simulink model "CRPNeuralNetwrok"  (R2019b)
settings: Solver=ode45  StartTime=0.0  StopTime=5  FixedStep=0.01  MaxStep=0.05  RelTol=1e-3
settings Model: Creator=user  LastModifiedBy=xyh
settings SolverCC: AlgebraicLoopSolver=LineSearch

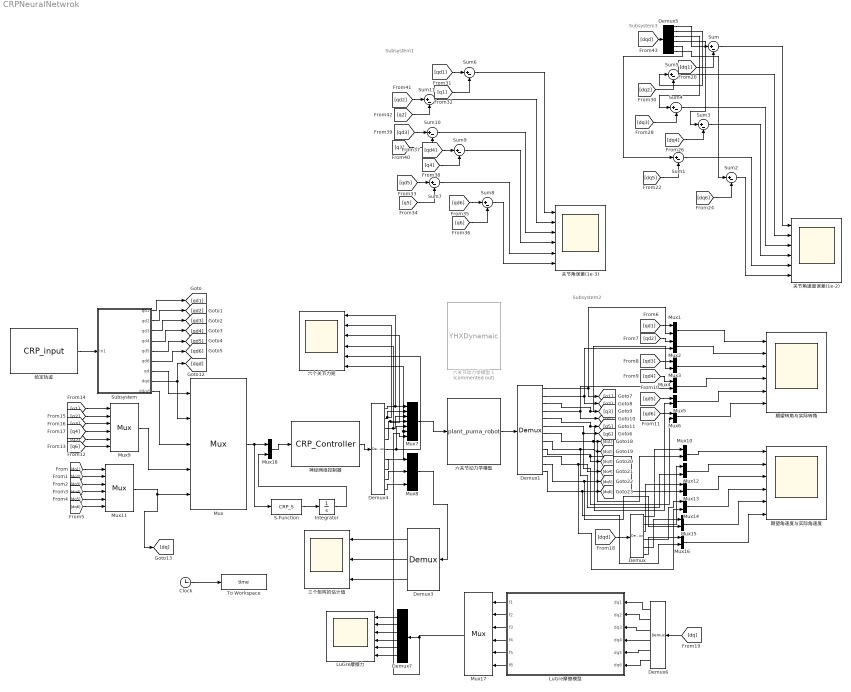
== system CRPNeuralNetwrok ==
  note: Subsystem1
  note: Subsystem3
  note: Subsystem2
  Clock : Clock
  Demux{,5..7} (4 alike) : Demux  Outputs=6
  Demux1 : Demux  Outputs=12
  Demux3 : Demux  Outputs=3
  Demux4 : Demux  Outputs=9
  Integrator : Integrator
  LuGre摩擦力 : Scope  NumInputPorts=6
  LuGre摩擦模型 : Subsystem
  Mux : Mux  Inputs=5
  Mux{1..6,10,12..16,18} (13 alike) : Mux  Inputs=2
  Mux11 : Mux  Inputs=6
  Mux17 : Mux  Inputs=6
  Mux7 : Mux  Inputs=7
  Mux8 : Mux  Inputs=3
  Mux9 : Mux  Inputs=6
  S-Function : S-Function  FunctionName=CRP_S  SFunctionDeploymentMode=off  EnableBusSupport=off
  Subsystem : Subsystem  TreatAsAtomicUnit=on
  Sum{,1..11} (12 alike) : Sum  Inputs=|+-
  To Workspace : ToWorkspace  VariableName=time  SaveFormat=Timeseries  SampleTime=-1
  三个矩阵的估计值 : Scope  NumInputPorts=3
  六个关节力矩 : Scope  NumInputPorts=6
  "六关节动力学模型 " : S-Function  FunctionName=plant_puma_robot  SFunctionDeploymentMode=off  EnableBusSupport=off
  六关节动力学模型 1 : S-Function  Commented=on  FunctionName=YHXDynamaic  SFunctionDeploymentMode=off  EnableBusSupport=off
  关节角误差(1e-3) : Scope  NumInputPorts=6
  关节角速度误差(1e-2) : Scope  NumInputPorts=6
  期望角速度与实际角速度 : Scope  NumInputPorts=6
  期望转角与实际转角 : Scope  NumInputPorts=6
  神经网络控制器 : S-Function  FunctionName=CRP_Controller  SFunctionDeploymentMode=off  EnableBusSupport=off
  给定轨迹 : S-Function  FunctionName=CRP_input  SFunctionDeploymentMode=off  EnableBusSupport=off
  wires:
  Mux7/1 -> "六关节动力学模型 "/1
  Clock/1 -> To Workspace/1
  [dq1] -> Mux11/1
  [dq4] -> Mux11/4
  [dq2] -> Mux11/2
  [dq3] -> Mux11/3
  [dq5] -> Mux11/5
  [dq6] -> Mux11/6
  Demux3/1 -> 三个矩阵的估计值/1
  Demux3/2 -> 三个矩阵的估计值/2
  Demux3/3 -> 三个矩阵的估计值/3
  神经网络控制器/1 -> Demux4/1
  Mux8/1 -> Demux3/1
  [q1] -> Mux9/1
  [q2] -> Mux9/2
  [q3] -> Mux9/3
  [q4] -> Mux9/4
  [q5] -> Mux9/5
  [q6] -> Mux9/6
  "六关节动力学模型 "/1 -> Demux1/1
  Demux4/3 -> 六个关节力矩/4, Mux7/3
  Demux4/1 -> 六个关节力矩/1, Mux7/1
  Demux4/2 -> 六个关节力矩/2, Mux7/2
  Demux4/4 -> 六个关节力矩/3, Mux7/4
  Demux4/5 -> 六个关节力矩/5, Mux7/5
  Demux4/6 -> 六个关节力矩/6, Mux7/6
  Demux4/7 -> Mux8/1
  Demux4/8 -> Mux8/2
  Demux4/9 -> Mux8/3
  Mux/1 -> S-Function/1, Mux18/1
  Mux11/1 -> [dq], Mux/5
  Mux9/1 -> Mux/4
  给定轨迹/1 -> Subsystem/1(In1)
  Subsystem/7(qd) -> Mux/1
  Subsystem/8(dqd) -> [dqd], Mux/2
  Subsystem/9(ddqd) -> Mux/3
  Subsystem/1(qd1) -> [qd1]
  Subsystem/2(qd2) -> [qd2]
  Subsystem/3(qd3) -> [qd3]
  Subsystem/4(qd4) -> [qd4]
  Subsystem/5(qd5) -> [qd5]
  Subsystem/6(qd6) -> [qd6]
  Sum6/1 -> 关节角误差(1e-3)/1
  Sum11/1 -> 关节角误差(1e-3)/2
  Sum10/1 -> 关节角误差(1e-3)/3
  Sum9/1 -> 关节角误差(1e-3)/4
  Sum7/1 -> 关节角误差(1e-3)/5
  Sum8/1 -> 关节角误差(1e-3)/6
  Mux1/1 -> 期望转角与实际转角/1
  Mux2/1 -> 期望转角与实际转角/2
  Mux3/1 -> 期望转角与实际转角/3
  Mux4/1 -> 期望转角与实际转角/4
  Mux5/1 -> 期望转角与实际转角/5
  Mux6/1 -> 期望转角与实际转角/6
  Mux10/1 -> 期望角速度与实际角速度/1
  Mux12/1 -> 期望角速度与实际角速度/2
  Mux13/1 -> 期望角速度与实际角速度/3
  Mux14/1 -> 期望角速度与实际角速度/4
  Mux15/1 -> 期望角速度与实际角速度/5
  Mux16/1 -> 期望角速度与实际角速度/6
  Demux/4 -> Mux14/1
  Demux1/12 -> Mux16/2, [dq6]
  Demux1/2 -> [q2], Mux2/2
  [qd2] -> Mux2/1
  Demux1/4 -> Mux4/2, [q4]
  [qd1] -> Mux1/1
  Demux/3 -> Mux13/1
  Demux1/1 -> [q1], Mux1/2
  Demux/6 -> Mux16/1
  Demux1/10 -> Mux14/2, [dq4]
  Demux/5 -> Mux15/1
  Demux/1 -> Mux10/1
  Demux1/9 -> Mux13/2, [dq3]
  [dqd] -> Demux/1
  [qd6] -> Mux6/1
  Demux1/7 -> Mux10/2, [dq1]
  [qd3] -> Mux3/1
  Demux1/11 -> [dq5], Mux15/2
  [qd4] -> Mux4/1
  [qd5] -> Mux5/1
  Demux1/5 -> Mux5/2, [q5]
  Demux/2 -> Mux12/1
  Demux1/6 -> Mux6/2, [q6]
  Demux1/8 -> Mux12/2, [dq2]
  Demux1/3 -> Mux3/2, [q3]
  Sum/1 -> 关节角速度误差(1e-2)/1
  Sum5/1 -> 关节角速度误差(1e-2)/2
  Sum4/1 -> 关节角速度误差(1e-2)/3
  Sum3/1 -> 关节角速度误差(1e-2)/4
  Sum1/1 -> 关节角速度误差(1e-2)/5
  Sum2/1 -> 关节角速度误差(1e-2)/6
  [dq2] -> Sum5/2
  Demux5/4 -> Sum3/1
  Demux5/5 -> Sum1/1
  Demux5/3 -> Sum4/1
  [dq5] -> Sum1/2
  Demux5/1 -> Sum/1
  [dq6] -> Sum2/2
  Demux5/6 -> Sum2/1
  Demux5/2 -> Sum5/1
  [dq3] -> Sum4/2
  [dq4] -> Sum3/2
  [dq1] -> Sum/2
  [q5] -> Sum7/2
  [qd1] -> Sum6/1
  [qd2] -> Sum11/1
  [q4] -> Sum9/2
  [qd3] -> Sum10/1
  [qd4] -> Sum9/1
  [q3] -> Sum10/2
  [qd5] -> Sum7/1
  [q6] -> Sum8/2
  [qd6] -> Sum8/1
  [q2] -> Sum11/2
  [q1] -> Sum6/2
  [dqd] -> Demux5/1
  LuGre摩擦模型/1(f1) -> Mux17/1
  LuGre摩擦模型/2(f2) -> Mux17/2
  LuGre摩擦模型/3(f3) -> Mux17/3
  LuGre摩擦模型/4(f4) -> Mux17/4
  LuGre摩擦模型/5(f5) -> Mux17/5
  LuGre摩擦模型/6(f6) -> Mux17/6
  [dq] -> Demux6/1
  Demux6/1 -> LuGre摩擦模型/1(dq1)
  Demux6/2 -> LuGre摩擦模型/2(dq2)
  Demux6/3 -> LuGre摩擦模型/3(dq3)
  Demux6/4 -> LuGre摩擦模型/4(dq4)
  Demux6/5 -> LuGre摩擦模型/5(dq5)
  Demux6/6 -> LuGre摩擦模型/6(dq6)
  Mux17/1 -> Mux7/7, Demux7/1
  Demux7/1 -> LuGre摩擦力/1
  Demux7/3 -> LuGre摩擦力/3
  Demux7/4 -> LuGre摩擦力/4
  Demux7/5 -> LuGre摩擦力/5
  Demux7/6 -> LuGre摩擦力/6
  Demux7/2 -> LuGre摩擦力/2
  S-Function/1 -> Integrator/1
  Mux18/1 -> 神经网络控制器/1
  Integrator/1 -> Mux18/2

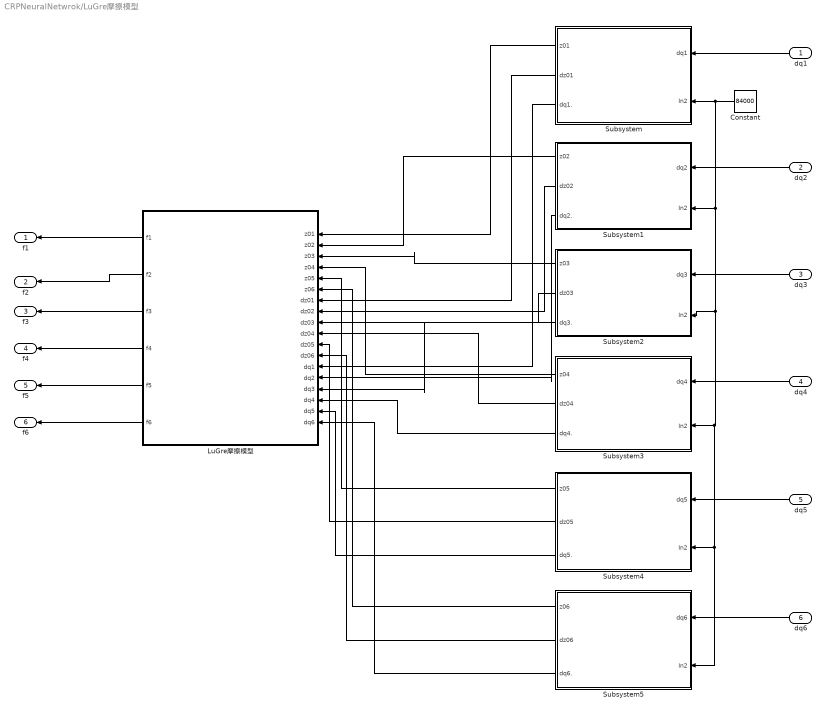
== system CRPNeuralNetwrok/LuGre摩擦模型 ==
  dq1 : Inport
  dq2 : Inport  Port=2
  dq3 : Inport  Port=3
  dq4 : Inport  Port=4
  dq5 : Inport  Port=5
  dq6 : Inport  Port=6
  Constant : Constant  Value=84000
  LuGre摩擦模型 : MATLAB Function  TreatAsAtomicUnit=on
  Subsystem : Subsystem
  Subsystem1 : Subsystem
  Subsystem2 : Subsystem
  Subsystem3 : Subsystem
  Subsystem4 : Subsystem
  Subsystem5 : Subsystem
  f1 : Outport
  f2 : Outport  Port=2
  f3 : Outport  Port=3
  f4 : Outport  Port=4
  f5 : Outport  Port=5
  f6 : Outport  Port=6
  wires:
  LuGre摩擦模型/2(f2) -> f2/1
  LuGre摩擦模型/1(f1) -> f1/1
  Constant/1 -> Subsystem5/2(In2), Subsystem4/2(In2), Subsystem3/2(In2), Subsystem2/2(In2), Subsystem1/2(In2), Subsystem/2(In2)
  dq1/1 -> Subsystem/1(dq1)
  Subsystem/1(z01) -> LuGre摩擦模型/1(z01)
  Subsystem/2(dz01) -> LuGre摩擦模型/7(dz01)
  Subsystem/3(dq1.) -> LuGre摩擦模型/13(dq1)
  dq2/1 -> Subsystem1/1(dq2)
  dq3/1 -> Subsystem2/1(dq3)
  dq4/1 -> Subsystem3/1(dq4)
  dq5/1 -> Subsystem4/1(dq5)
  dq6/1 -> Subsystem5/1(dq6)
  Subsystem1/1(z02) -> LuGre摩擦模型/2(z02)
  Subsystem1/2(dz02) -> LuGre摩擦模型/8(dz02)
  Subsystem1/3(dq2.) -> LuGre摩擦模型/14(dq2)
  Subsystem2/1(z03) -> LuGre摩擦模型/3(z03)
  Subsystem2/2(dz03) -> LuGre摩擦模型/9(dz03)
  Subsystem2/3(dq3.) -> LuGre摩擦模型/15(dq3)
  Subsystem3/1(z04) -> LuGre摩擦模型/4(z04)
  Subsystem3/2(dz04) -> LuGre摩擦模型/10(dz04)
  Subsystem3/3(dq4.) -> LuGre摩擦模型/16(dq4)
  Subsystem4/1(z05) -> LuGre摩擦模型/5(z05)
  Subsystem4/2(dz05) -> LuGre摩擦模型/11(dz05)
  Subsystem4/3(dq5.) -> LuGre摩擦模型/17(dq5)
  Subsystem5/1(z06) -> LuGre摩擦模型/6(z06)
  Subsystem5/2(dz06) -> LuGre摩擦模型/12(dz06)
  Subsystem5/3(dq6.) -> LuGre摩擦模型/18(dq6)
  LuGre摩擦模型/6(f6) -> f6/1
  LuGre摩擦模型/5(f5) -> f5/1
  LuGre摩擦模型/4(f4) -> f4/1
  LuGre摩擦模型/3(f3) -> f3/1

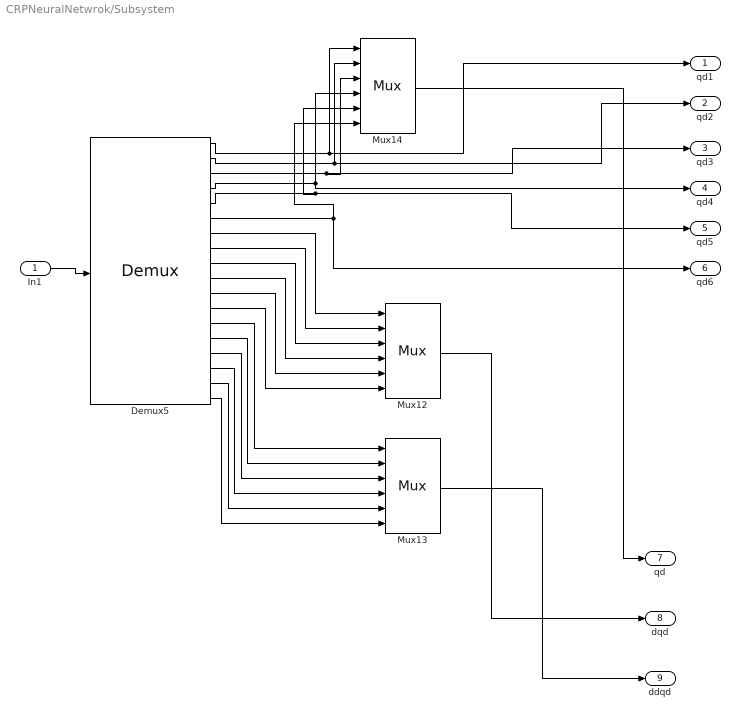
== system CRPNeuralNetwrok/Subsystem ==
  In1 : Inport
  Demux5 : Demux  Outputs=18
  Mux12 : Mux  Inputs=6
  Mux13 : Mux  Inputs=6
  Mux14 : Mux  Inputs=6
  qd1 : Outport
  qd2 : Outport  Port=2
  qd3 : Outport  Port=3
  qd4 : Outport  Port=4
  qd5 : Outport  Port=5
  qd6 : Outport  Port=6
  qd : Outport  Port=7
  dqd : Outport  Port=8
  ddqd : Outport  Port=9
  wires:
  Demux5/8 -> Mux12/2
  Demux5/2 -> Mux14/2, qd2/1
  Demux5/3 -> Mux14/3, qd3/1
  Mux13/1 -> ddqd/1
  Demux5/11 -> Mux12/5
  Demux5/4 -> qd4/1, Mux14/4
  Demux5/1 -> Mux14/1, qd1/1
  Demux5/5 -> Mux14/5, qd5/1
  Demux5/13 -> Mux13/1
  In1/1 -> Demux5/1
  Demux5/7 -> Mux12/1
  Demux5/6 -> Mux14/6, qd6/1
  Mux12/1 -> dqd/1
  Demux5/12 -> Mux12/6
  Demux5/14 -> Mux13/2
  Demux5/18 -> Mux13/6
  Demux5/16 -> Mux13/4
  Mux14/1 -> qd/1
  Demux5/17 -> Mux13/5
  Demux5/10 -> Mux12/4
  Demux5/9 -> Mux12/3
  Demux5/15 -> Mux13/3

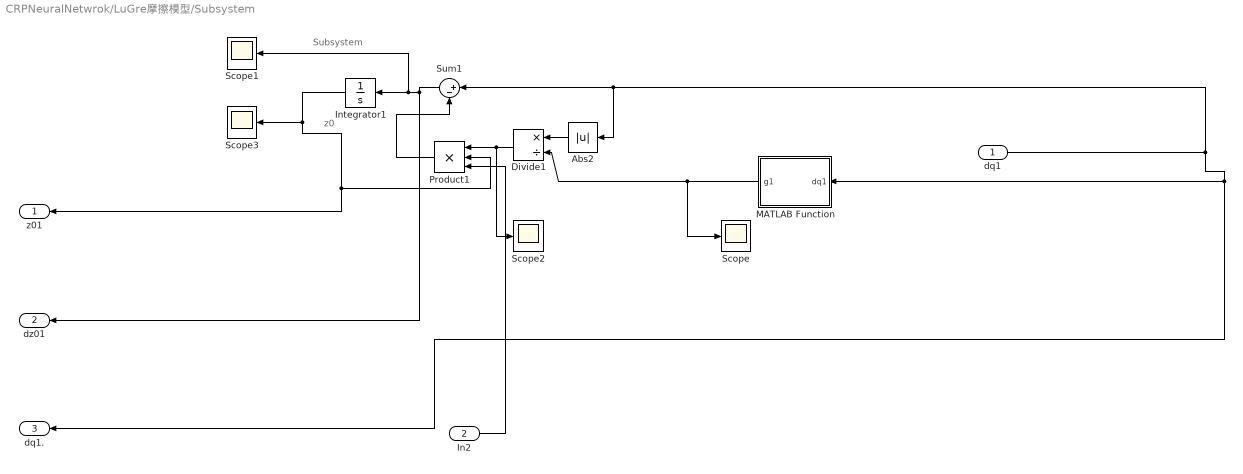
== system CRPNeuralNetwrok/LuGre摩擦模型/Subsystem ==
  note: z0
  note: Subsystem
  dq1 : Inport
  In2 : Inport  Port=2
  Abs2 : Abs
  Divide1 : Product  Inputs=*/
  Integrator1 : Integrator
  MATLAB Function : MATLAB Function  TreatAsAtomicUnit=on
  Product1 : Product  Inputs=3
  Scope{,1..3} (4 alike) : Scope
  Sum1 : Sum  Inputs=|+-
  z01 : Outport
  dz01 : Outport  Port=2
  dq1. : Outport  Port=3
  wires:
  Product1/1 -> Sum1/2
  Abs2/1 -> Divide1/1
  Integrator1/1 -> Scope3/1, z01/1, Product1/2
  Sum1/1 -> dz01/1, Scope1/1, Integrator1/1
  Divide1/1 -> Product1/1, Scope2/1
  dq1/1 -> Abs2/1, Sum1/1, dq1./1, MATLAB Function/1(dq1)
  In2/1 -> Product1/3
  MATLAB Function/1(g1) -> Divide1/2, Scope/1

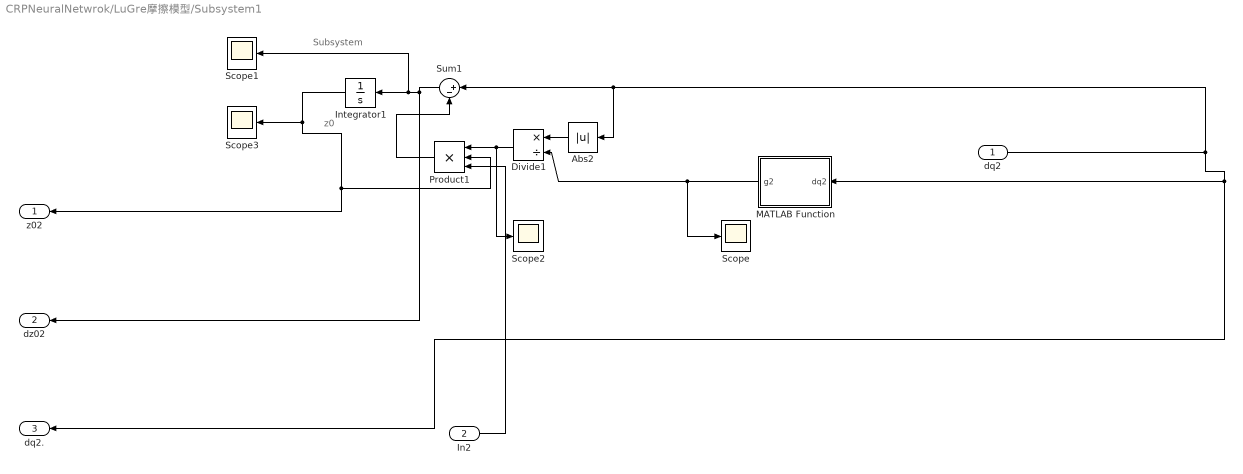
== system CRPNeuralNetwrok/LuGre摩擦模型/Subsystem1 ==
  note: Subsystem
  note: z0
  dq2 : Inport
  In2 : Inport  Port=2
  Abs2 : Abs
  Divide1 : Product  Inputs=*/
  Integrator1 : Integrator
  MATLAB Function : MATLAB Function  TreatAsAtomicUnit=on
  Product1 : Product  Inputs=3
  Scope{,1..3} (4 alike) : Scope
  Sum1 : Sum  Inputs=|+-
  z02 : Outport
  dz02 : Outport  Port=2
  dq2. : Outport  Port=3
  wires:
  MATLAB Function/1(g2) -> Scope/1, Divide1/2
  In2/1 -> Product1/3
  dq2/1 -> MATLAB Function/1(dq2), dq2./1, Sum1/1, Abs2/1
  Divide1/1 -> Scope2/1, Product1/1
  Sum1/1 -> Integrator1/1, Scope1/1, dz02/1
  Integrator1/1 -> Product1/2, z02/1, Scope3/1
  Abs2/1 -> Divide1/1
  Product1/1 -> Sum1/2

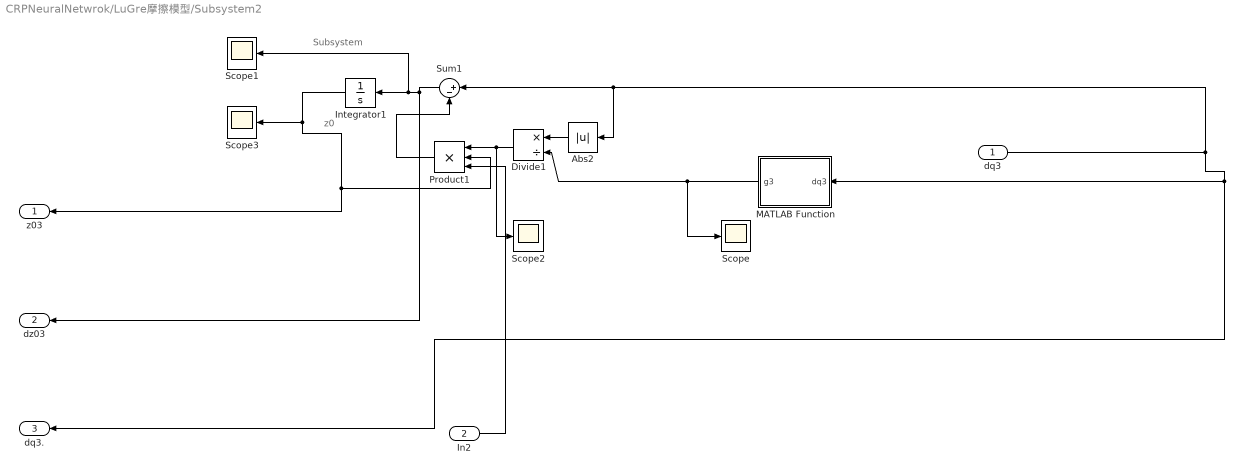
== system CRPNeuralNetwrok/LuGre摩擦模型/Subsystem2 ==
  note: z0
  note: Subsystem
  dq3 : Inport
  In2 : Inport  Port=2
  Abs2 : Abs
  Divide1 : Product  Inputs=*/
  Integrator1 : Integrator
  MATLAB Function : MATLAB Function  TreatAsAtomicUnit=on
  Product1 : Product  Inputs=3
  Scope{,1..3} (4 alike) : Scope
  Sum1 : Sum  Inputs=|+-
  z03 : Outport
  dz03 : Outport  Port=2
  dq3. : Outport  Port=3
  wires:
  Product1/1 -> Sum1/2
  Abs2/1 -> Divide1/1
  Integrator1/1 -> Scope3/1, z03/1, Product1/2
  Sum1/1 -> dz03/1, Scope1/1, Integrator1/1
  Divide1/1 -> Product1/1, Scope2/1
  dq3/1 -> Abs2/1, Sum1/1, dq3./1, MATLAB Function/1(dq3)
  In2/1 -> Product1/3
  MATLAB Function/1(g3) -> Divide1/2, Scope/1

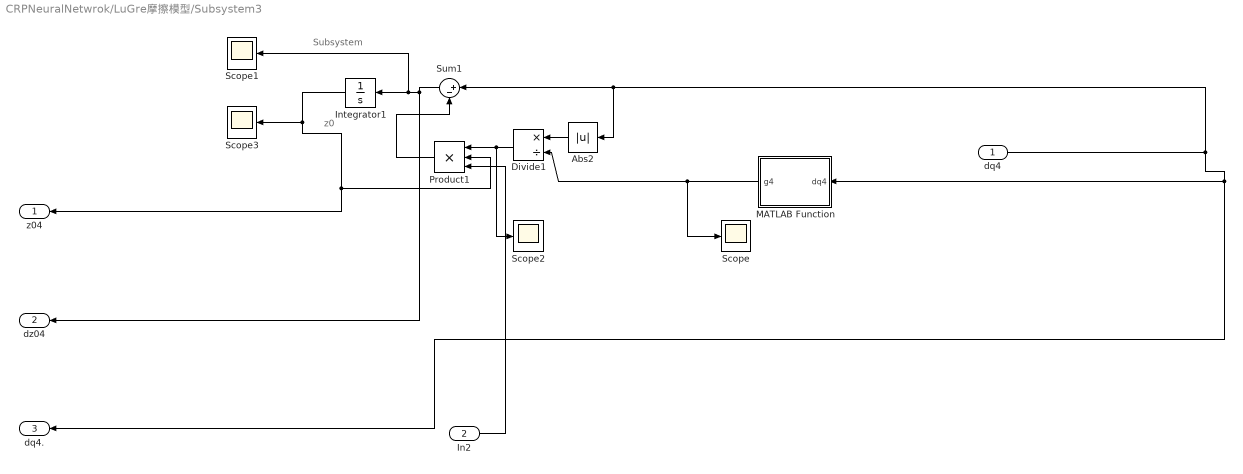
== system CRPNeuralNetwrok/LuGre摩擦模型/Subsystem3 ==
  note: Subsystem
  note: z0
  dq4 : Inport
  In2 : Inport  Port=2
  Abs2 : Abs
  Divide1 : Product  Inputs=*/
  Integrator1 : Integrator
  MATLAB Function : MATLAB Function  TreatAsAtomicUnit=on
  Product1 : Product  Inputs=3
  Scope{,1..3} (4 alike) : Scope
  Sum1 : Sum  Inputs=|+-
  z04 : Outport
  dz04 : Outport  Port=2
  dq4. : Outport  Port=3
  wires:
  MATLAB Function/1(g4) -> Scope/1, Divide1/2
  In2/1 -> Product1/3
  dq4/1 -> MATLAB Function/1(dq4), dq4./1, Sum1/1, Abs2/1
  Divide1/1 -> Scope2/1, Product1/1
  Sum1/1 -> Integrator1/1, Scope1/1, dz04/1
  Integrator1/1 -> Product1/2, z04/1, Scope3/1
  Abs2/1 -> Divide1/1
  Product1/1 -> Sum1/2

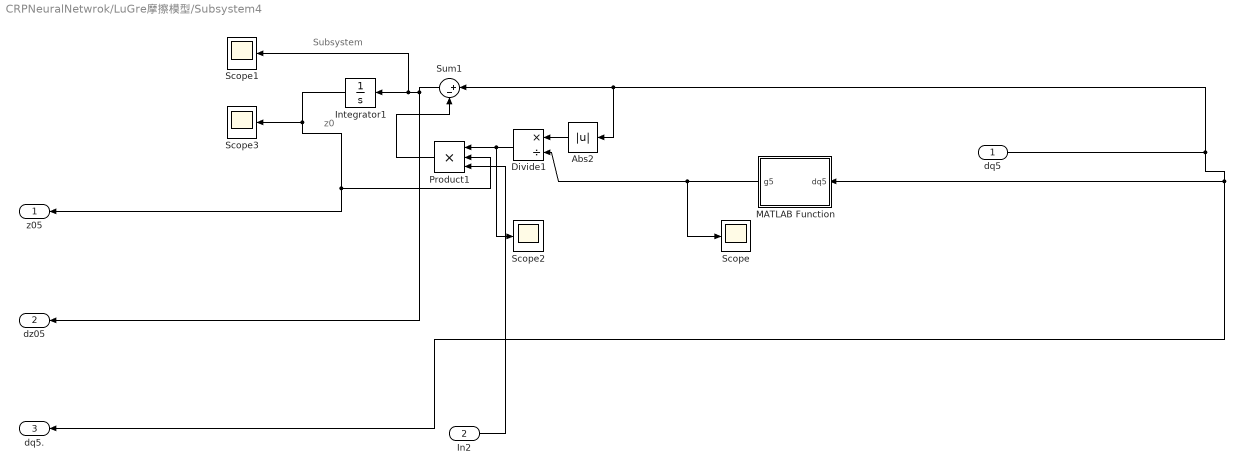
== system CRPNeuralNetwrok/LuGre摩擦模型/Subsystem4 ==
  note: z0
  note: Subsystem
  dq5 : Inport
  In2 : Inport  Port=2
  Abs2 : Abs
  Divide1 : Product  Inputs=*/
  Integrator1 : Integrator
  MATLAB Function : MATLAB Function  TreatAsAtomicUnit=on
  Product1 : Product  Inputs=3
  Scope{,1..3} (4 alike) : Scope
  Sum1 : Sum  Inputs=|+-
  z05 : Outport
  dz05 : Outport  Port=2
  dq5. : Outport  Port=3
  wires:
  Product1/1 -> Sum1/2
  Abs2/1 -> Divide1/1
  Integrator1/1 -> Scope3/1, z05/1, Product1/2
  Sum1/1 -> dz05/1, Scope1/1, Integrator1/1
  Divide1/1 -> Product1/1, Scope2/1
  dq5/1 -> Abs2/1, Sum1/1, dq5./1, MATLAB Function/1(dq5)
  In2/1 -> Product1/3
  MATLAB Function/1(g5) -> Divide1/2, Scope/1

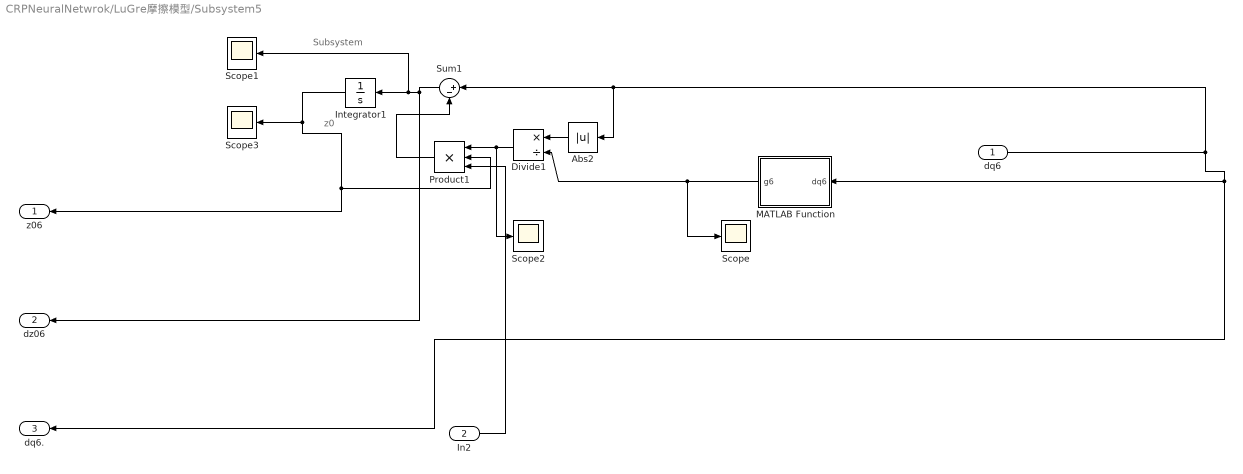
== system CRPNeuralNetwrok/LuGre摩擦模型/Subsystem5 ==
  note: Subsystem
  note: z0
  dq6 : Inport
  In2 : Inport  Port=2
  Abs2 : Abs
  Divide1 : Product  Inputs=*/
  Integrator1 : Integrator
  MATLAB Function : MATLAB Function  TreatAsAtomicUnit=on
  Product1 : Product  Inputs=3
  Scope{,1..3} (4 alike) : Scope
  Sum1 : Sum  Inputs=|+-
  z06 : Outport
  dz06 : Outport  Port=2
  dq6. : Outport  Port=3
  wires:
  MATLAB Function/1(g6) -> Scope/1, Divide1/2
  In2/1 -> Product1/3
  dq6/1 -> MATLAB Function/1(dq6), dq6./1, Sum1/1, Abs2/1
  Divide1/1 -> Scope2/1, Product1/1
  Sum1/1 -> Integrator1/1, Scope1/1, dz06/1
  Integrator1/1 -> Product1/2, z06/1, Scope3/1
  Abs2/1 -> Divide1/1
  Product1/1 -> Sum1/2

== matlab function CRPNeuralNetwrok/LuGre摩擦模型/Subsystem1/MATLAB Function ==
  data: dq2 input; g2 output
function g2 = fcn(dq2)
xite1 = 260;
xite2 = 28;
Fc = 3.82;
Fs = 8.16;
dqs = 0.0125;

g2 = Fc + (Fs-Fc)*exp(-(dq2/dqs)^2);

== matlab function CRPNeuralNetwrok/LuGre摩擦模型/Subsystem2/MATLAB Function ==
  data: dq3 input; g3 output
function g3 = fcn(dq3)
xite1 = 260;
xite2 = 28;
Fc = 3.82;
Fs = 8.16;
dqs = 0.0125;

g3 = Fc + (Fs-Fc)*exp(-(dq3/dqs)^2);

== matlab function CRPNeuralNetwrok/LuGre摩擦模型/Subsystem3/MATLAB Function ==
  data: dq4 input; g4 output
function g4 = fcn(dq4)
xite1 = 260;
xite2 = 28;
Fc = 3.82;
Fs = 8.16;
dqs = 0.0125;

g4 = Fc + (Fs-Fc)*exp(-(dq4/dqs)^2);

== matlab function CRPNeuralNetwrok/LuGre摩擦模型/Subsystem4/MATLAB Function ==
  data: dq5 input; g5 output
function g5 = fcn(dq5)
xite1 = 260;
xite2 = 28;
Fc = 3.82;
Fs = 8.16;
dqs = 0.0125;

g5 = Fc + (Fs-Fc)*exp(-(dq5/dqs)^2);

== matlab function CRPNeuralNetwrok/LuGre摩擦模型/Subsystem5/MATLAB Function ==
  data: dq6 input; g6 output
function g6 = fcn(dq6)
xite1 = 260;
xite2 = 28;
Fc = 3.82;
Fs = 8.16;
dqs = 0.0125;

g6 = Fc + (Fs-Fc)*exp(-(dq6/dqs)^2);

== matlab function CRPNeuralNetwrok/LuGre摩擦模型/LuGre摩擦模型 ==
  data: z01 input; z02 input; z03 input; z04 input; z05 input; z06 input; dz01 input; dz02 input; dz03 input; dz04 input; dz05 input; dz06 input; dq1 input; f1 output; dq2 input; f2 output; f3 output; f4 output; f5 output; f6 output; dq3 input; dq4 input; dq5 input; dq6 input
function [f1,f2,f3,f4,f5,f6] = fcn(z01,z02,z03,z04,z05,z06,dz01,dz02,dz03,dz04,dz05,dz06,dq1,dq2,dq3,dq4,dq5,dq6)
xite0 = 84000;
xite1 = 260;
xite2 = 28;
Fc = 3.82;
Fs = 8.16;
dqs = 0.0125;
lamda = 1;

f1 = lamda * (xite0 * z01 + xite1 * dz01 + xite2 * dq1);
f2 = lamda * (xite0 * z02 + xite1 * dz02 + xite2 * dq2);
f3 = lamda * (xite0 * z03 + xite1 * dz03 + xite2 * dq3);
f4 = lamda * (xite0 * z04 + xite1 * dz04 + xite2 * dq4);
f5 = lamda * (xite0 * z05 + xite1 * dz05 + xite2 * dq5);
f6 = lamda * (xite0 * z06 + xite1 * dz06 + xite2 * dq6);

== matlab function CRPNeuralNetwrok/LuGre摩擦模型/Subsystem/MATLAB Function ==
  data: dq1 input; g1 output
function g1 = fcn(dq1)
xite1 = 260;
xite2 = 28;
Fc = 3.82;
Fs = 8.16;
dqs = 0.0125;

g1 = Fc + (Fs-Fc)*exp(-(dq1/dqs)^2);
